simulink model "VSP"  (Simulink 7.7)
settings: Solver=ode45  StartTime=0.0  StopTime=50e-3  RelTol=1e-3
values from neighbouring files (symbols this model uses):
  ki = (wn^2)/Em    [PLL_Init_3approaches.m]    (also in PLL_Init_complete_without_recent_errata.m; approach_comp.m = (wn.^2)./Em; cardan_self_consistent.m; cardan_self_consistent_inbuiltsolve.m)
  kp = 2*del*wn/Em    [PLL_Init_3approaches.m]    (also in PLL_Init_complete_without_recent_errata.m; approach_comp.m = 2.*del.*wn/Em; cardan_self_consistent.m; cardan_self_consistent_inbuiltsolve.m)
libraries: simulink_extras x1, aerolibobsolete x1
settings Model: Creator=Sambhav  LastModifiedBy=Sambhav

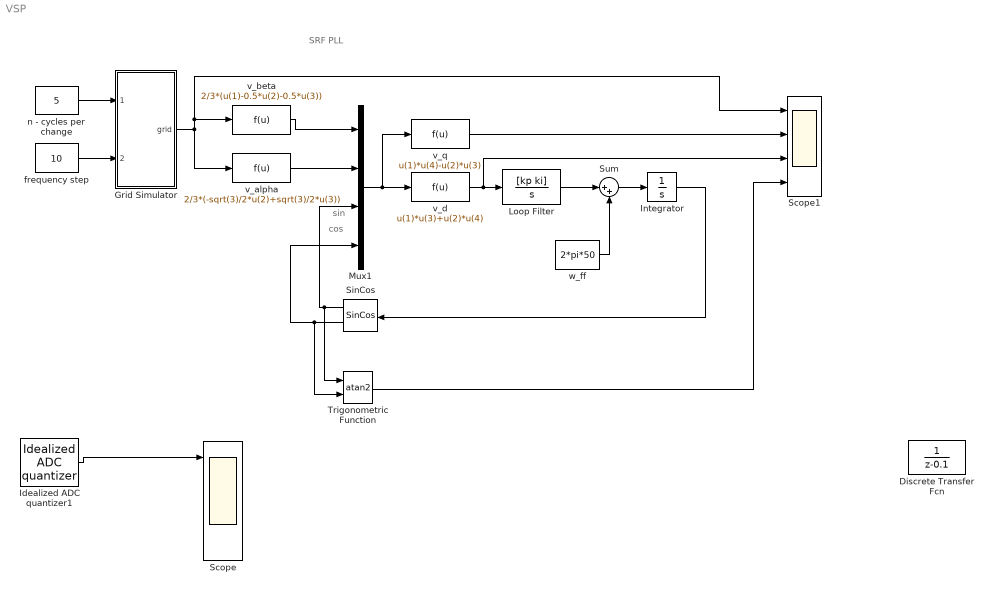
== system VSP ==
  note: sin
  note: cos
  note: SRF PLL
  Discrete Transfer Fcn : DiscreteTransferFcn  Denominator=[1 -0.1]
  Grid Simulator : Subsystem
  Idealized ADC quantizer1 : simulink_extras/Additional Discrete/Idealized ADC quantizer  SystemSampleTime=-1  NumberOfConverterBits=4  Vmin=-240*sqrt(2)  Vmax=240*sqrt(2)  OutputDataType=int16  OutputNegativeValues=on
  Integrator : Integrator
  Loop Filter : TransferFcn  Numerator=[kp ki]  Denominator=[1 0]
  Mux1 : Mux
  Scope : Scope  NumInputPorts=4
      settings: TimeRange=0.8  YMin=-500~-4~294.8412698412699~-60  YMax=500~4~362.3015873015872~20  SampleInput=on  SampleTime=0.0001
  Scope1 : Scope  NumInputPorts=4
      settings: YMin=-5~-5~-5~-5  YMax=5~5~5~5  SampleInput=on  SampleTime=0.0001
  SinCos : aerolibobsolete/SinCos  SystemSampleTime=-1
  Sum : Sum  Inputs=|++
  Trigonometric Function : Trigonometry  Operator=atan2
  frequency step : Constant  Value=10
  n - cycles per change : Constant  Value=5
  v_alpha : Fcn  Expr=2/3*(-sqrt(3)/2*u(2)+sqrt(3)/2*u(3))
  v_beta : Fcn  Expr=2/3*(u(1)-0.5*u(2)-0.5*u(3))
  v_d : Fcn  Expr=u(1)*u(3)+u(2)*u(4)
  v_q : Fcn  Expr=u(1)*u(4)-u(2)*u(3)
  w_ff : Constant  Value=2*pi*50
  wires:
  n - cycles per change/1 -> Grid Simulator/1(n cycles)
  frequency step/1 -> Grid Simulator/2(freq_step)
  Idealized ADC quantizer1/1 -> Scope/1
  Loop Filter/1 -> Sum/1
  w_ff/1 -> Sum/2
  Sum/1 -> Integrator/1
  v_d/1 -> Loop Filter/1, Scope1/3
  Integrator/1 -> SinCos/1
  Mux1/1 -> v_d/1, v_q/1
  SinCos/2 -> Mux1/4, Trigonometric Function/2
  SinCos/1 -> Mux1/3, Trigonometric Function/1
  v_alpha/1 -> Mux1/2
  v_beta/1 -> Mux1/1
  v_q/1 -> Scope1/2
  Trigonometric Function/1 -> Scope1/4
  Grid Simulator/1(grid) -> v_alpha/1, Scope1/1, v_beta/1

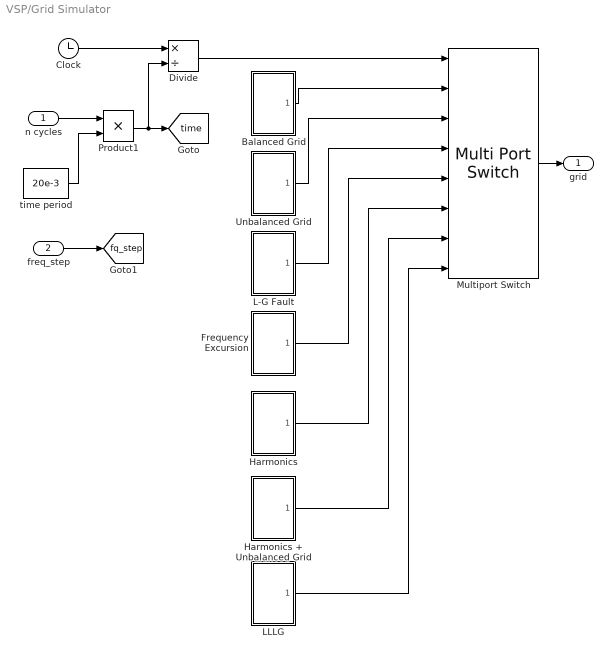
== system VSP/Grid Simulator ==
  n cycles : Inport
  freq_step : Inport  Port=2
  Balanced Grid : Subsystem
  Clock : Clock
  Divide : Product  Inputs=*/
  Frequency Excursion : Subsystem
  Harmonics : Subsystem
  Harmonics + Unbalanced Grid : Subsystem
  L-G Fault : Subsystem
  LLLG : Subsystem
  Multiport Switch : MultiPortSwitch  Inputs=7  DiagnosticForDefault=None  zeroidx=off
  Product1 : Product  RndMeth=Zero
  Unbalanced Grid : Subsystem
  time period : Constant  Value=20e-3
  grid : Outport
  tag scope: fq_step=global, time=global
  wires:
  Unbalanced Grid/1(v_grid) -> Multiport Switch/3
  Balanced Grid/1(v_grid) -> Multiport Switch/2
  L-G Fault/1(v_grid) -> Multiport Switch/4
  Frequency Excursion/1(v_grid) -> Multiport Switch/5
  Harmonics/1(v_grid) -> Multiport Switch/6
  Clock/1 -> Divide/1
  time period/1 -> Product1/2
  Product1/1 -> Divide/2, [time]
  Divide/1 -> Multiport Switch/1
  LLLG/1(v_grid) -> Multiport Switch/8
  Harmonics + Unbalanced Grid/1(v_grid) -> Multiport Switch/7
  n cycles/1 -> Product1/1
  Multiport Switch/1 -> grid/1
  freq_step/1 -> [fq_step]

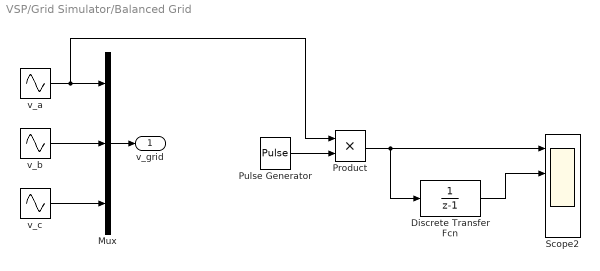
== system VSP/Grid Simulator/Balanced Grid ==
  Discrete Transfer Fcn : DiscreteTransferFcn  Denominator=[1 -1]  SampleTime=0.0001
  Mux : Mux  Inputs=3
  Product : Product  RndMeth=Zero
  Pulse Generator : DiscretePulseGenerator  PulseType=Time based  Period=1e-3  PulseWidth=1e-10
  Scope2 : Scope  NumInputPorts=4
      settings: YMin=-5~-5~-5~-5  YMax=5~5~5~5  SaveName=ScopeData2  SampleInput=on  SampleTime=0.0001
  v_a : Sin  Amplitude=230*sqrt(2)  Frequency=2*pi*50  Phase=pi/2  SampleTime=0
  v_b : Sin  Amplitude=230*sqrt(2)  Frequency=2*pi*50  Phase=pi/2-2*pi/3  SampleTime=0
  v_c : Sin  Amplitude=230*sqrt(2)  Frequency=2*pi*50  Phase=pi/2+2*pi/3  SampleTime=0
  v_grid : Outport
  wires:
  v_a/1 -> Mux/1, Product/1
  v_b/1 -> Mux/2
  v_c/1 -> Mux/3
  Mux/1 -> v_grid/1
  Product/1 -> Scope2/1, Discrete Transfer Fcn/1
  Pulse Generator/1 -> Product/2
  Discrete Transfer Fcn/1 -> Scope2/2

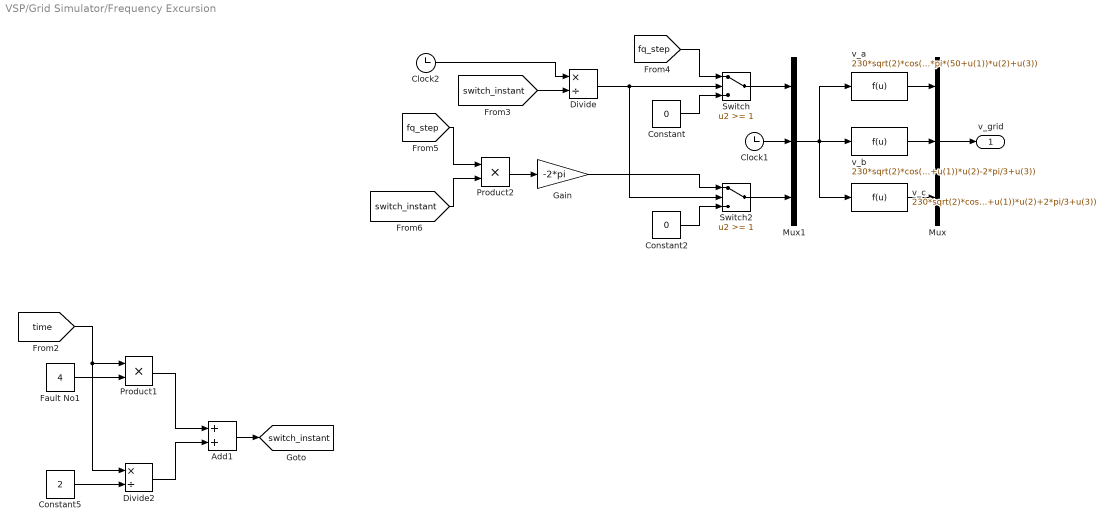
== system VSP/Grid Simulator/Frequency Excursion ==
  Add1 : Sum
  Clock1 : Clock
      settings: Decimation=10
  Clock2 : Clock
      settings: Decimation=10
  Constant : Constant  Value=0
  Constant2 : Constant  Value=0
  Constant5 : Constant  Value=2
  Divide : Product  Inputs=*/
  Divide2 : Product  Inputs=*/
  Fault No1 : Constant  Value=4
  Gain : Gain  Gain=-2*pi
  Mux : Mux  Inputs=3
  Mux1 : Mux  Inputs=3
  Product1 : Product  RndMeth=Zero
  Product2 : Product  RndMeth=Zero
  Switch : Switch  Threshold=1
  Switch2 : Switch  Threshold=1
  v_a : Fcn  Expr=230*sqrt(2)*cos(2*pi*(50+u(1))*u(2)+u(3))
  v_b : Fcn  Expr=230*sqrt(2)*cos(2*pi*(50+u(1))*u(2)-2*pi/3+u(3))
  v_c : Fcn  Expr=230*sqrt(2)*cos(2*pi*(50+u(1))*u(2)+2*pi/3+u(3))
  v_grid : Outport
  tag scope: switch_instant=global
  wires:
  [fq_step] -> Switch/1
  Constant/1 -> Switch/3
  Mux1/1 -> v_a/1, v_b/1, v_c/1
  v_a/1 -> Mux/1
  v_b/1 -> Mux/2
  v_c/1 -> Mux/3
  Constant2/1 -> Switch2/3
  Switch2/1 -> Mux1/3
  Gain/1 -> Switch2/1
  [time] -> Divide2/1, Product1/1
  Fault No1/1 -> Product1/2
  Product1/1 -> Add1/1
  Constant5/1 -> Divide2/2
  Divide2/1 -> Add1/2
  Mux/1 -> v_grid/1
  Switch/1 -> Mux1/1
  Clock2/1 -> Divide/1
  Add1/1 -> [switch_instant]
  [switch_instant] -> Divide/2
  Divide/1 -> Switch/2, Switch2/2
  [fq_step] -> Product2/1
  [switch_instant] -> Product2/2
  Product2/1 -> Gain/1
  Clock1/1 -> Mux1/2

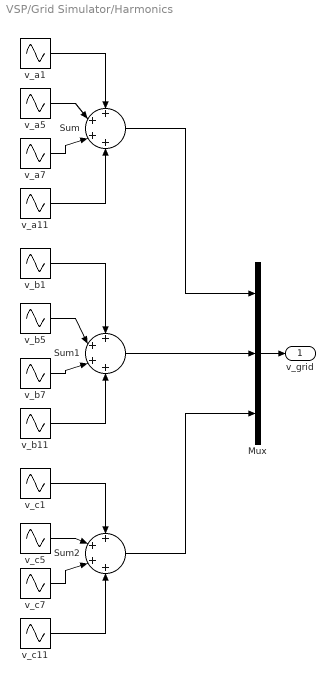
== system VSP/Grid Simulator/Harmonics ==
  Mux : Mux  Inputs=3
  Sum : Sum  Inputs=+|+|+|+
  Sum1 : Sum  Inputs=+|+|+|+
  Sum2 : Sum  Inputs=+|+|+|+
  v_a1 : Sin  Amplitude=230*sqrt(2)  Frequency=2*pi*50  Phase=pi/2  SampleTime=0
  v_a11 : Sin  Amplitude=230*sqrt(2)/11  Frequency=2*pi*50*11  Phase=pi/2  SampleTime=0
  v_a5 : Sin  Amplitude=230*sqrt(2)/5  Frequency=2*pi*50*5  Phase=pi/2  SampleTime=0
  v_a7 : Sin  Amplitude=230*sqrt(2)/7  Frequency=2*pi*50*7  Phase=pi/2  SampleTime=0
  v_b1 : Sin  Amplitude=230*sqrt(2)  Frequency=2*pi*50  Phase=pi/2-2*pi/3  SampleTime=0
  v_b11 : Sin  Amplitude=230*sqrt(2)/11  Frequency=2*pi*50*11  Phase=pi/2-2*pi/3  SampleTime=0
  v_b5 : Sin  Amplitude=230*sqrt(2)/5  Frequency=2*pi*50*5  Phase=pi/2-2*pi/3  SampleTime=0
  v_b7 : Sin  Amplitude=230*sqrt(2)/7  Frequency=2*pi*50*7  Phase=pi/2-2*pi/3  SampleTime=0
  v_c1 : Sin  Amplitude=230*sqrt(2)  Frequency=2*pi*50  Phase=pi/2+2*pi/3  SampleTime=0
  v_c11 : Sin  Amplitude=230*sqrt(2)/11  Frequency=2*pi*50*11  Phase=pi/2+2*pi/3  SampleTime=0
  v_c5 : Sin  Amplitude=230*sqrt(2)/5  Frequency=2*pi*50*5  Phase=pi/2+2*pi/3  SampleTime=0
  v_c7 : Sin  Amplitude=230*sqrt(2)/7  Frequency=2*pi*50*7  Phase=pi/2+2*pi/3  SampleTime=0
  v_grid : Outport
  wires:
  Mux/1 -> v_grid/1
  v_a1/1 -> Sum/1
  v_a5/1 -> Sum/2
  v_a7/1 -> Sum/3
  v_a11/1 -> Sum/4
  v_b1/1 -> Sum1/1
  v_b11/1 -> Sum1/4
  v_b5/1 -> Sum1/2
  v_b7/1 -> Sum1/3
  v_c1/1 -> Sum2/1
  v_c5/1 -> Sum2/2
  v_c7/1 -> Sum2/3
  v_c11/1 -> Sum2/4
  Sum/1 -> Mux/1
  Sum1/1 -> Mux/2
  Sum2/1 -> Mux/3

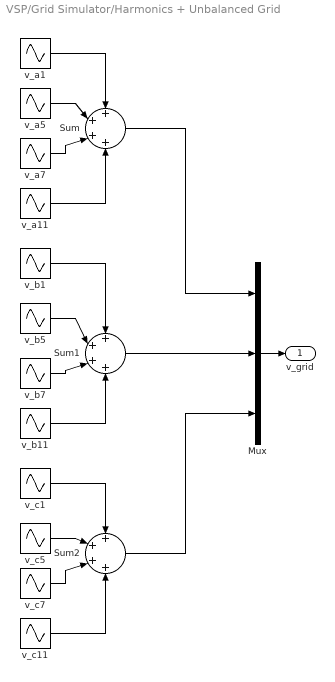
== system VSP/Grid Simulator/Harmonics + Unbalanced Grid ==
  Mux : Mux  Inputs=3
  Sum : Sum  Inputs=+|+|+|+
  Sum1 : Sum  Inputs=+|+|+|+
  Sum2 : Sum  Inputs=+|+|+|+
  v_a1 : Sin  Amplitude=230*sqrt(2)  Frequency=2*pi*50  Phase=pi/2  SampleTime=0
  v_a11 : Sin  Amplitude=230*sqrt(2)/11  Frequency=2*pi*50*11  Phase=pi/2  SampleTime=0
  v_a5 : Sin  Amplitude=230*sqrt(2)/5  Frequency=2*pi*50*5  Phase=pi/2  SampleTime=0
  v_a7 : Sin  Amplitude=230*sqrt(2)/7  Frequency=2*pi*50*7  Phase=pi/2  SampleTime=0
  v_b1 : Sin  Amplitude=200*sqrt(2)  Frequency=2*pi*50  Phase=pi/2-2*pi/3+pi/6  SampleTime=0
  v_b11 : Sin  Amplitude=220*sqrt(2)/11  Frequency=2*pi*50*11  Phase=pi/2-2*pi/3+pi/6  SampleTime=0
  v_b5 : Sin  Amplitude=200*sqrt(2)/5  Frequency=2*pi*50*5  Phase=pi/2-2*pi/3+pi/6  SampleTime=0
  v_b7 : Sin  Amplitude=200*sqrt(2)/7  Frequency=2*pi*50*7  Phase=pi/2-2*pi/3+pi/6  SampleTime=0
  v_c1 : Sin  Amplitude=210*sqrt(2)  Frequency=2*pi*50  Phase=pi/2+2*pi/3-pi/18  SampleTime=0
  v_c11 : Sin  Amplitude=210*sqrt(2)/11  Frequency=2*pi*50*11  Phase=pi/2+2*pi/3-pi/18  SampleTime=0
  v_c5 : Sin  Amplitude=210*sqrt(2)/5  Frequency=2*pi*50*5  Phase=pi/2+2*pi/3-pi/18  SampleTime=0
  v_c7 : Sin  Amplitude=210*sqrt(2)/7  Frequency=2*pi*50*7  Phase=pi/2+2*pi/3-pi/18  SampleTime=0
  v_grid : Outport
  wires:
  Sum2/1 -> Mux/3
  Sum1/1 -> Mux/2
  Sum/1 -> Mux/1
  v_c11/1 -> Sum2/4
  v_c7/1 -> Sum2/3
  v_c5/1 -> Sum2/2
  v_c1/1 -> Sum2/1
  v_b7/1 -> Sum1/3
  v_b5/1 -> Sum1/2
  v_b11/1 -> Sum1/4
  v_b1/1 -> Sum1/1
  v_a11/1 -> Sum/4
  v_a7/1 -> Sum/3
  v_a5/1 -> Sum/2
  v_a1/1 -> Sum/1
  Mux/1 -> v_grid/1

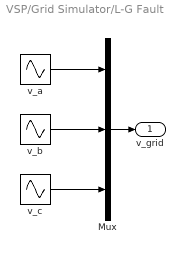
== system VSP/Grid Simulator/L-G Fault ==
  Mux : Mux  Inputs=3
  v_a : Sin  Amplitude=230*sqrt(2)  Frequency=2*pi*50  Phase=pi/2  SampleTime=0
  v_b : Sin  Amplitude=10  Frequency=2*pi*50  Phase=pi/2-2*pi/3  SampleTime=0
  v_c : Sin  Amplitude=230*sqrt(2)  Frequency=2*pi*50  Phase=pi/2+2*pi/3  SampleTime=0
  v_grid : Outport
  wires:
  Mux/1 -> v_grid/1
  v_c/1 -> Mux/3
  v_b/1 -> Mux/2
  v_a/1 -> Mux/1

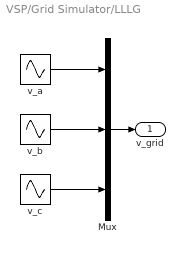
== system VSP/Grid Simulator/LLLG ==
  Mux : Mux  Inputs=3
  v_a : Sin  Amplitude=0  Frequency=0  SampleTime=0
  v_b : Sin  Amplitude=0  Frequency=0  SampleTime=0
  v_c : Sin  Amplitude=0  Frequency=0  SampleTime=0
  v_grid : Outport
  wires:
  Mux/1 -> v_grid/1
  v_c/1 -> Mux/3
  v_b/1 -> Mux/2
  v_a/1 -> Mux/1

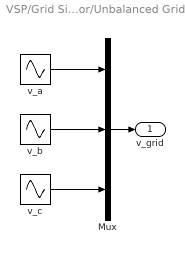
== system VSP/Grid Simulator/Unbalanced Grid ==
  Mux : Mux  Inputs=3
  v_a : Sin  Amplitude=230*sqrt(2)  Frequency=2*pi*50  Phase=pi/2  SampleTime=0
  v_b : Sin  Amplitude=200*sqrt(2)  Frequency=2*pi*50  Phase=pi/2-2*pi/3+pi/6  SampleTime=0
  v_c : Sin  Amplitude=210*sqrt(2)  Frequency=2*pi*50  Phase=pi/2+2*pi/3-pi/18  SampleTime=0
  v_grid : Outport
  wires:
  v_a/1 -> Mux/1
  v_b/1 -> Mux/2
  v_c/1 -> Mux/3
  Mux/1 -> v_grid/1
